simulink model "msdDoubleSimulationOutput"  (R2020b)
settings: Solver=VariableStepAuto  StartTime=0.0  StopTime=20  RelTol=1e-6
settings Model: Creator=Rocksmithed  LastModifiedBy=Rocksmithed
settings DataIOCC: SaveFormat=Array

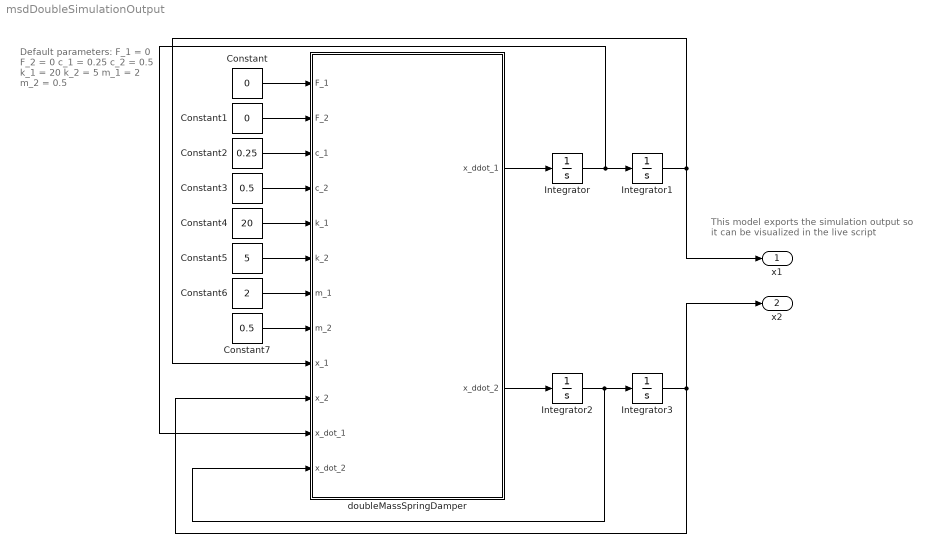
== system msdDoubleSimulationOutput ==
  note: Default parameters:
      |
      | F_1 = 0
      | F_2 = 0
      | c_1 = 0.25
      | c_2 = 0.5
      | k_1 = 20
      | k_2 = 5
      | m_1 = 2
      | m_2 = 0.5
  note: This model exports the simulation output
      | so it can be visualized in the live script
  Constant : Constant  Value=0
  Constant1 : Constant  Value=0
  Constant2 : Constant  Value=0.25
  Constant3 : Constant  Value=0.5
  Constant4 : Constant  Value=20
  Constant5 : Constant  Value=5
  Constant6 : Constant  Value=2
  Constant7 : Constant  Value=0.5
  Integrator : Integrator
  Integrator1 : Integrator
  Integrator2 : Integrator  InitialCondition=8
  Integrator3 : Integrator
  doubleMassSpringDamper : MATLAB Function  TreatAsAtomicUnit=on
  x1 : Outport
  x2 : Outport  Port=2
  wires:
  Constant/1 -> doubleMassSpringDamper/1(F_1)
  Constant1/1 -> doubleMassSpringDamper/2(F_2)
  Constant2/1 -> doubleMassSpringDamper/3(c_1)
  Constant3/1 -> doubleMassSpringDamper/4(c_2)
  Constant4/1 -> doubleMassSpringDamper/5(k_1)
  Constant5/1 -> doubleMassSpringDamper/6(k_2)
  Constant6/1 -> doubleMassSpringDamper/7(m_1)
  Constant7/1 -> doubleMassSpringDamper/8(m_2)
  doubleMassSpringDamper/1(x_ddot_1) -> Integrator/1
  Integrator/1 -> doubleMassSpringDamper/11(x_dot_1), Integrator1/1
  doubleMassSpringDamper/2(x_ddot_2) -> Integrator2/1
  Integrator2/1 -> doubleMassSpringDamper/12(x_dot_2), Integrator3/1
  Integrator1/1 -> x1/1, doubleMassSpringDamper/9(x_1)
  Integrator3/1 -> x2/1, doubleMassSpringDamper/10(x_2)

== matlab function msdDoubleSimulationOutput/doubleMassSpringDamper ==
  data: F_1 input; x_ddot_1 output; F_2 input; c_1 input; c_2 input; k_1 input; k_2 input; m_1 input; m_2 input; x_1 input; x_2 input; x_dot_1 input; x_dot_2 input; x_ddot_2 output
function [x_ddot_1,x_ddot_2] = doubleMassSpringDamper(F_1,F_2,c_1,c_2,k_1,k_2,m_1,m_2,x_1,x_2,x_dot_1,x_dot_2)
%#codegen

%    This function was generated by the Symbolic Math Toolbox version 8.6.
%    12-Nov-2020 14:51:47

t2 = -x_2;
t3 = -x_dot_2;
t4 = t2+x_1;
t5 = t3+x_dot_1;
t6 = c_2.*t5;
t7 = k_2.*t4;
x_ddot_1 = -(-F_1+t6+t7+c_1.*x_dot_1+k_1.*x_1)./m_1;
if nargout > 1
    x_ddot_2 = (F_2+t6+t7)./m_2;
end
